simulink model "Task1Ab"  (R2024a)
settings: Solver=VariableStepAuto  StartTime=0.0  StopTime=10.0  RelTol=1e-3
undefined symbols (not defined in the file): b, k, m
settings Model: Creator=kyleo  LastModifiedBy=kyleo

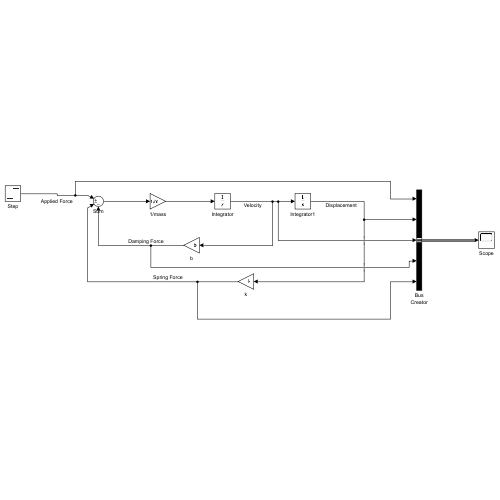
[thumbnail: Simulink's stored preview of the top-level diagram]
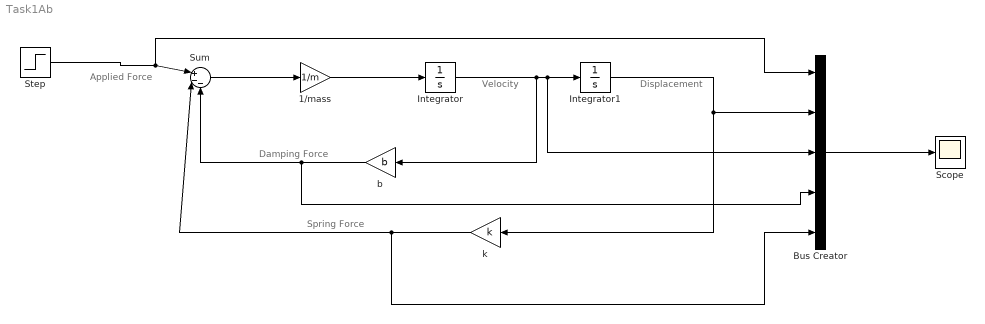
== system Task1Ab ==
  note: Velocity
  note: Damping Force
  note: Displacement
  note: Applied Force
  note: Spring Force
  1/mass : Gain  Gain=1/m
  Bus Creator : BusCreator  Inputs=5
  Integrator : Integrator
  Integrator1 : Integrator
  Scope : Scope
  Step : Step  After=2  SampleTime=0
  Sum : Sum  Inputs=|+--
  b : Gain  Gain=b
  k : Gain  Gain=k
  wires:
  Step/1 -> Bus Creator/1, Sum/1
  b/1 -> Bus Creator/4, Sum/3
  k/1 -> Bus Creator/5, Sum/2
  Sum/1 -> 1/mass/1
  1/mass/1 -> Integrator/1
  Integrator/1 -> b/1, Bus Creator/3, Integrator1/1
  Integrator1/1 -> Bus Creator/2, k/1
  Bus Creator/1 -> Scope/1
